simulink model "ESTS_FRIC_HILO_PREPROC_test"  (R2024b)
settings: Solver=VariableStepAuto  StartTime=0.0  StopTime=10.0  RelTol=1e-3
libraries: ESTS_FRIC_HILO_PREPROC x1
settings Model: Creator=blatak  LastModifiedBy=blatak

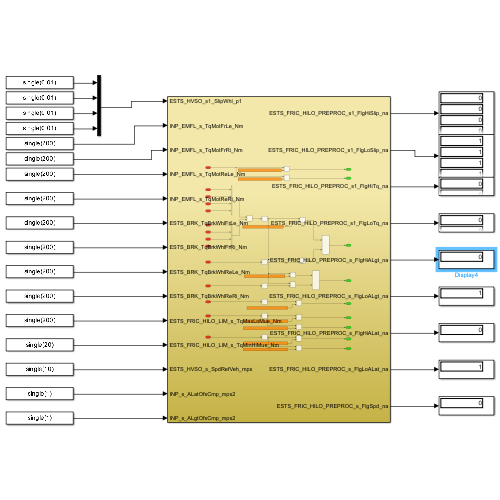
[thumbnail: Simulink's stored preview of the top-level diagram]
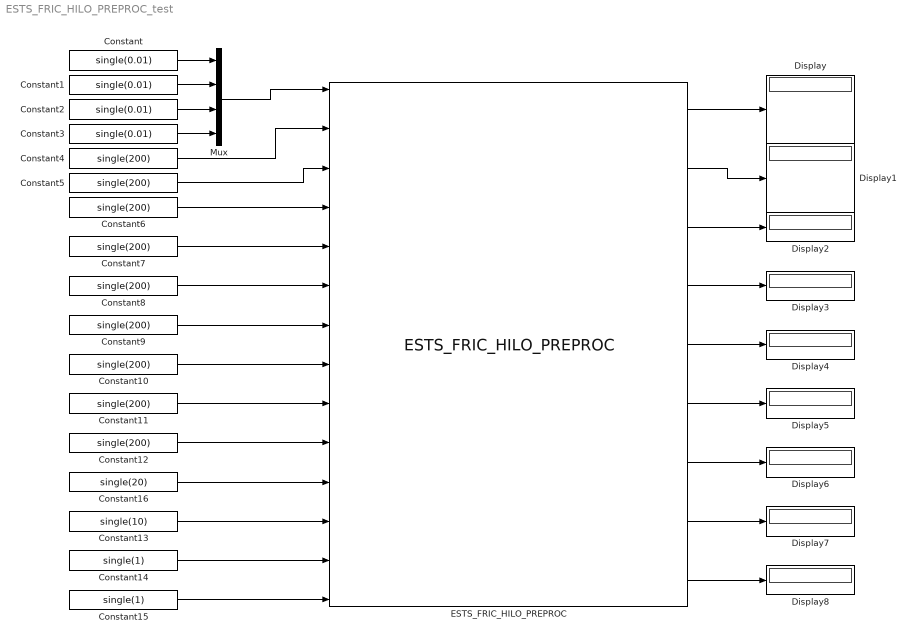
== system ESTS_FRIC_HILO_PREPROC_test ==
  Constant{,1..3} (4 alike) : Constant  Value=single(0.01)
  Constant{4..12} (9 alike) : Constant  Value=single(200)
  Constant13 : Constant  Value=single(10)
  Constant14 : Constant  Value=single(1)
  Constant15 : Constant  Value=single(1)
  Constant16 : Constant  Value=single(20)
  Display{,1..8} (9 alike) : Display
  ESTS_FRIC_HILO_PREPROC : ESTS_FRIC_HILO_PREPROC/ESTS_FRIC_HILO_PREPROC  SystemSampleTime=-1  VariantActivationTime=update diagram  AllowFlexibleInterface=on  Latency=0  AutoFrameSizeCalculation=off
  Mux : Mux
  wires:
  Constant/1 -> Mux/1
  Constant1/1 -> Mux/2
  Constant2/1 -> Mux/3
  Constant3/1 -> Mux/4
  Mux/1 -> ESTS_FRIC_HILO_PREPROC/1
  Constant4/1 -> ESTS_FRIC_HILO_PREPROC/2
  Constant5/1 -> ESTS_FRIC_HILO_PREPROC/3
  Constant6/1 -> ESTS_FRIC_HILO_PREPROC/4
  Constant7/1 -> ESTS_FRIC_HILO_PREPROC/5
  Constant8/1 -> ESTS_FRIC_HILO_PREPROC/6
  Constant9/1 -> ESTS_FRIC_HILO_PREPROC/7
  Constant10/1 -> ESTS_FRIC_HILO_PREPROC/8
  Constant11/1 -> ESTS_FRIC_HILO_PREPROC/9
  Constant12/1 -> ESTS_FRIC_HILO_PREPROC/10
  Constant13/1 -> ESTS_FRIC_HILO_PREPROC/12
  Constant14/1 -> ESTS_FRIC_HILO_PREPROC/13
  Constant15/1 -> ESTS_FRIC_HILO_PREPROC/14
  Constant16/1 -> ESTS_FRIC_HILO_PREPROC/11
  ESTS_FRIC_HILO_PREPROC/1 -> Display/1
  ESTS_FRIC_HILO_PREPROC/2 -> Display1/1
  ESTS_FRIC_HILO_PREPROC/3 -> Display2/1
  ESTS_FRIC_HILO_PREPROC/4 -> Display3/1
  ESTS_FRIC_HILO_PREPROC/5 -> Display4/1
  ESTS_FRIC_HILO_PREPROC/6 -> Display5/1
  ESTS_FRIC_HILO_PREPROC/7 -> Display6/1
  ESTS_FRIC_HILO_PREPROC/8 -> Display7/1
  ESTS_FRIC_HILO_PREPROC/9 -> Display8/1
